simulink model "s3"  (Simulink 2.00)
settings: Solver=ode45  StartTime=0.0  StopTime=tstop  MaxStep=0.01  RelTol=1e-5  AbsTol=1e-6
values from neighbouring files (symbols this model uses):
  iLo = 0    [M2.M]    (also in M2INIT.M; M3.M; M4.M)
  L = 0.1    [M2.M]    (also in M2INIT.M; M3.M = 0.04; M4.M = 0.000231)
  R = 0.4    [M3.M]    (also in M4.M = 12)
  Vac_mag = 100    [M3.M]
  we = 314    [M3.M]    (also in M4.M = (0.5*wo: 0.01*wo: 1.5*wo))
settings Model: SaveTime=off  SaveOutput=off  ConsistencyChecking=off

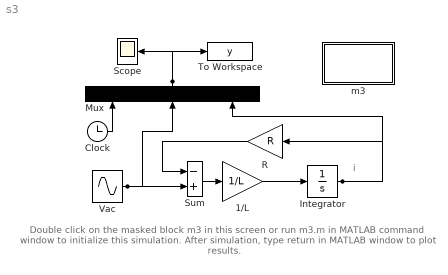
== system s3 ==
  note: i
  note: Double click on the masked block m3 in this screen or run m3.m
      | in MATLAB command window to initialize this simulation.
      | After simulation,  type return in MATLAB window to plot results.
  1/L : Gain  Gain=1/L
  Clock : Clock
      settings: DeleteFcn=simclock BlockIsBeingDestroyed  PostSaveFcn=simclock Save
  m3 : Subsystem
      settings: OpenFcn=m3
      mask Type: Masked block of m3.m
      mask Help: Uses m3.m to initialize
      mask Display: disp('Initialize\nm3SIM')
  Integrator : Integrator  ExternalReset=none  InitialConditionSource=internal  InitialCondition=iLo  LimitOutput=off  UpperSaturationLimit=inf  LowerSaturationLimit=-inf  ShowSaturationPort=off  ShowStatePort=off  AbsoluteTolerance=auto
  Mux : Mux  Orientation=up  Inputs=3
  R : Gain  Orientation=left  Gain=R
  Scope : Scope
      settings: TickLabels=on  TimeRange=auto  YMin=-100  YMax=100  SaveToWorkspace=off  SaveName=ScopeData
  Sum : Sum  Inputs=-+
  To Workspace : ToWorkspace  VariableName=y  SampleTime=0
      settings: Buffer=3000
  Vac : Sin  Amplitude=Vac_mag  Frequency=we  Phase=0  SampleTime=-1
  wires:
  Integrator/1 -> Mux/3, R/1
  Vac/1 -> Mux/2, Sum/2
  R/1 -> Sum/1
  Sum/1 -> 1/L/1
  Mux/1 -> Scope/1, To Workspace/1
  Clock/1 -> Mux/1
  1/L/1 -> Integrator/1

== system s3/m3 ==
  note: Masked block of m3.m to initialize
      | and plot results
